simulink model "x15_model"  (R2015a)
settings: Solver=ode3  SolverMode=SingleTasking  StartTime=t_s  StopTime=t_e  FixedStep=dt  RelTol=1e-3
undefined symbols (not defined in the file): A, B, C, D, dt, init
settings Model: CovMetricSettings=dwe  covSaveCumulativeToWorkspaceVar=off  CovSaveSingleToWorkspaceVar=off  CovExternalEMLEnable=on  Creator=yakov  LastModifiedBy=79534
settings DataIOCC: LimitDataPoints=off  SaveFormat=Dataset  ReturnWorkspaceOutputs=on
settings OptimizationCC: InlineParams=on  OptimizeModelRefInitCode=on
settings DebuggingCC: SFUnexpectedBacktrackingDiag=error  SFNoUnconditionalDefaultTransitionDiag=error
settings HardwareCC: ProdBitPerPointer=64  ProdLargestAtomicFloat=Float  ProdIntDivRoundTo=Zero  ProdEndianess=LittleEndian  ProdHWDeviceType=Specified  TargetBitPerPointer=64  TargetLongLongMode=on  TargetIntDivRoundTo=Zero  TargetEndianess=LittleEndian  TargetWordSize=64  TargetHWDeviceType=MATLAB Host  ProdEqTarget=off
settings ModelReferenceCC: PropagateSignalLabelsOutOfModel=on
settings SFSimCC: SimUseLocalCustomCode=on
settings RTWCC: Description=Embedded Coder (host-based shared library target)  SystemTargetFile=ert_shrlib.tlc  GenCodeOnly=on  TemplateMakefile=ert_default_tmf  RTWUseLocalCustomCode=on
settings CodeAppCC: IgnoreCustomStorageClasses=off
settings STFCustomTargetCC: ParMdlRefBuildCompliant=on  CompOptLevelCompliant=on  CombineOutputUpdateFcns=on  SupportVariableSizeSignals=off  ModelStepFunctionPrototypeControlCompliant=on  SystemTargetFile=ert_shrlib.tlc
settings ERTTargetCC: ParMdlRefBuildCompliant=on  CompOptLevelCompliant=on  SupportVariableSizeSignals=off  ModelStepFunctionPrototypeControlCompliant=on  ERTCustomFileTemplate=example_file_process.tlc

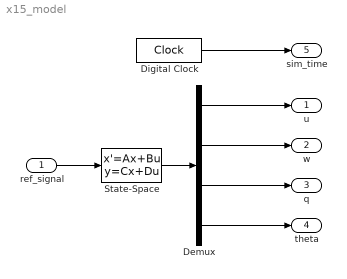
== system x15_model ==
  ref_signal : Inport
  Demux : Demux
  Digital Clock : DigitalClock  SampleTime=dt
  State-Space : StateSpace  A=A  B=B  C=C  D=D  X0=init  ContinuousStateAttributes={'u','w', 'q', 'theta'}
  u : Outport
  w : Outport  Port=2
  q : Outport  Port=3
  theta : Outport  Port=4
  "sim_time " : Outport  Port=5
  wires:
  ref_signal/1 -> State-Space/1
  Demux/2 -> w/1
  State-Space/1 -> Demux/1
  Demux/1 -> u/1
  Demux/3 -> q/1
  Demux/4 -> theta/1
  Digital Clock/1 -> "sim_time "/1
